simulink library "teme2eci_lib"  (R2018b)
settings: Solver=VariableStepAuto  StartTime=0.0  StopTime=10.0  RelTol=1e-3
settings Model: Creator=Kate  LastModifiedBy=Kate

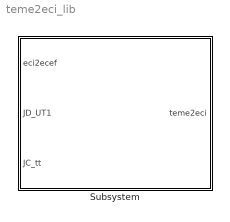
== system teme2eci_lib ==
  Subsystem : Subsystem

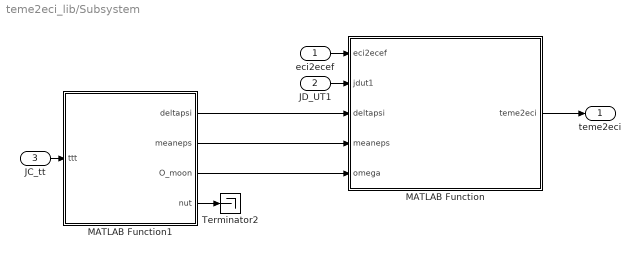
== system teme2eci_lib/Subsystem ==
  eci2ecef : Inport
  JD_UT1 : Inport  Port=2
  JC_tt : Inport  Port=3
  MATLAB Function : MATLAB Function  TreatAsAtomicUnit=on
  MATLAB Function1 : MATLAB Function  TreatAsAtomicUnit=on
  Terminator2 : Terminator
  teme2eci : Outport
  wires:
  MATLAB Function1/1(deltapsi) -> MATLAB Function/3(deltapsi)
  MATLAB Function1/4(nut) -> Terminator2/1
  eci2ecef/1 -> MATLAB Function/1(eci2ecef)
  JD_UT1/1 -> MATLAB Function/2(jdut1)
  JC_tt/1 -> MATLAB Function1/1(ttt)
  MATLAB Function1/2(meaneps) -> MATLAB Function/4(meaneps)
  MATLAB Function1/3(O_moon) -> MATLAB Function/5(omega)
  MATLAB Function/1(teme2eci) -> teme2eci/1

== matlab function teme2eci_lib/Subsystem/MATLAB Function1 ==
  data: ttt input; deltapsi output; meaneps output; O_moon output; nut output
%Author Kate Williams
%Date 1/24/2019

%Last edit by Kate Williams 2/14/2019, changed method of final matrix to use rot1,rot3
%terms
%conversions
function [deltapsi, meaneps,O_moon,nut] = nutation(ttt)
        %OUTPUT ANGLES IN RADIANTS
        deg2rad = pi/180.0; %deg to rad
        rad2deg = 1/deg2rad;
        asec2rad = 1/3600*deg2rad;
        ttt2= ttt*ttt; %ttt is julian century in tt time frame
        ttt3= ttt2*ttt;
        
        %mean obliquity of the ecliptic in rads
        meaneps = deg2rad * ( 23.439291 ...
                        - 0.0130042 * ttt ...
                        - 1.64e-7 * ttt2 ...
                        + 5.04e-7 * ttt3);
                % ---- iau 1980 theory
% Largest Nutation coefficents (out of 106)                    
        nc = [ ...
            1   0   0   0   0   1   -171996 -174.2  92025   8.9
            9   0   0   2   -2  2   -13187  -1.6    5736    -3.1
            31  0   0   2   0   2   -2274   -0.2    977     -0.5
            2   0   0   0   0   2   2062    0.2     -895    0.5
            10  0   1   0  	0   0   1426    -3.4    54      -0.1
            32  1   0   0   0   0   712     0.1     -7      0.0
            11  0   1   2   -2  2   -517    1.2     224     -0.6
            33  0   0   2   0   1   -386    -0.4    200     0.0
            34  1   0   2   0   2   -301    0.0     129     -0.1
            12  0   -1  2   -2  2   217     -0.5    -95     0.3
            35  1   0   0   -2  0   -158    0.0     -1      0.0
            13  0   0   2   -2  1   129     0.1     -70     0.0 
            36  -1  0   2   0   2   123     0.0     -53     0.0 
            38  1   0   0   0   1   63      0.1     -33     0.0
            37  0   0   0   2   0   63      0.0     -2      0.0
            40  -1  0   2   2   2   -59     0.0     26      0.0
            39  -1  0   0   0   1   -58     -0.1    32      0.0
            41  1   0   2   0   1   -51     0.0     27      0.0
            14  2   0   0   -2  0   48      0.0     1       0.0
            3   -2  0   2   0   1   46      0.0     -24     0.0
            42  0   0   2   2   2   -38     0.0     16      0.0
            45  2   0   2   0   2   -31     0.0     13      0.0
            43  2   0   0   0   0   29      0.0     -1      0.0
            44  1   0   2   -2  2   29      0.0     -12     0.0
            46  0   0   2   0   0   26      0.0     -1      0.0
            15  0   0   2   -2  0   -22     0.0     0       0.0
            47  -1  0   2   0   1   21      0.0     -10     0.0
            16  0   2   0   0   0   17      -0.1    0       0.0
            18  0   2   2   -2  2   -16     0.1     7       0.0
            48  -1  0   0   2   1   16      0.0     -8      0.0 ...
            ];
        
        M_moon	=   deg2rad * ( 134.96298139+(1325 * 360 + 198.8673981) * ttt ...
                      	+ 0.0086972 * ttt2 + 1.78e-5 * ttt3);
               
        M_sun	=   deg2rad * ( 357.52772333 + (99 * 360 + 359.0503400) * ttt ...
                        - 0.0001603 * ttt2 - 3.3e-6 * ttt3);

        U_moon	=   deg2rad * ( 93.27191028 + (1342 * 360 + 82.0175381) * ttt ...
                        - 0.0036825 * ttt2 + 3.1e-6 * ttt3);

        D_sun	=   deg2rad * ( 297.85036306 + (1236 * 360 + 307.1114800) * ttt ...
                        - 0.0019142 * ttt^2 + 5.3e-6 *ttt^3);

        O_moon	=   deg2rad * ( 125.04452222 - (5 * 360 + 134.1362608) * ttt ...
                        + 0.0020708 * ttt^2 + 2.2e-6 * ttt^3);       
            
        % ---- ANGLES of nutation from equ 3-82 of vallado 
        M_moon    = rem( M_moon,360.0  )     * deg2rad; % rad %moon
        M_sun   = rem( M_sun,360.0  )    * deg2rad;%sun
        U_moon    = rem( U_moon,360.0  )     * deg2rad;%moon
        D_sun    = rem( D_sun,360.0  )     * deg2rad;%sun
        O_moon= rem( O_moon,360.0  ) * deg2rad;%moon
        
        %find nutation in longitude and nutation in obliquity
        deltapsi= 0.0; %nutation angle in rad set initially to zero
        deltaeps= 0.0; %change in obliquity in rad
        
        for i = 1:size(nc,1)
            tempval    =   nc(i,2) * M_moon + nc(i,3) * M_sun + nc(i,4) * U_moon + nc(i,5) * D_sun + nc(i,6) * O_moon;
            deltapsi   =   0.0001 * (nc(i,7) + nc(i,8) * ttt) * sin(tempval) + deltapsi;
            deltaeps   =   0.0001 * (nc(i,9) + nc(i,10) * ttt) * cos(tempval) + deltaeps;
        end

        
        %final nutation parameters, see page 226 equ. 3-85of Vallado
        trueeps  = meaneps + deltaeps*asec2rad; %true obliquity of eclipti

        %complete nutation rotation matrix
        nut=zeros(3,3);
        
        rot1_meaneps=[1 0 0;0 cos(-meaneps) sin(-meaneps);0 -sin(-meaneps) cos(-meaneps)];
        rot3_deltapsi=[cos(asec2rad * deltapsi) sin(asec2rad * deltapsi) 0;-sin(asec2rad * deltapsi) cos(asec2rad * deltapsi) 0;0 0 1];
        rot1_trueeps=[1 0 0;0 cos(trueeps) sin(trueeps);0 -sin(trueeps) cos(trueeps)];
        
        nut = rot1_meaneps* rot3_deltapsi* rot1_trueeps;   
        
         %testing THis must be kept. 
        deltapsi = deltapsi*asec2rad; 
        deltaeps = deltaeps*asec2rad;
end

== matlab function teme2eci_lib/Subsystem/MATLAB Function ==
  data: eci2ecef input; teme2eci output; jdut1 input; deltapsi input; meaneps input; omega input
function teme2eci  = TEME2ECI(eci2ecef,jdut1,deltapsi,meaneps,omega)
%polar motion neglected 

%INPUTS
%    eci2ecef    - transformation matrix eci - ecef
%    jdut1       - julian centuries of ut1        days
%    deltapsi    - nutation angle                 rad
%    meaneps     - mean obliquity of the ecliptic rad
%    omega       - long of asc node of moon       rad

%OUTPUTS
%    teme2eci    - transformation matrix teme - ecef

%locals        :
%    st          - matrix for pef - tod 


 %TEME to ecef

 %transformation matrix that accounts for the effects of sidereal time
 [st,stdot] = sidereal(jdut1,deltapsi,meaneps,omega);

 %rotation for polar motion (pef - ecef) assumed unity

 %TEME to ECEF to ECI
 
 teme2eci=st'*eci2ecef';

end
